simulink model "Quad_Joystick"  (R2018a)
settings: Solver=ode45  StartTime=0.0  StopTime=inf  RelTol=1e-3
undefined symbols (not defined in the file or in its folder): Q
libraries: vrlib x4, realtime_pacer_lib x1, sharedtransform x1
settings Model: Creator=Jarvis  LastModifiedBy=Jarvis

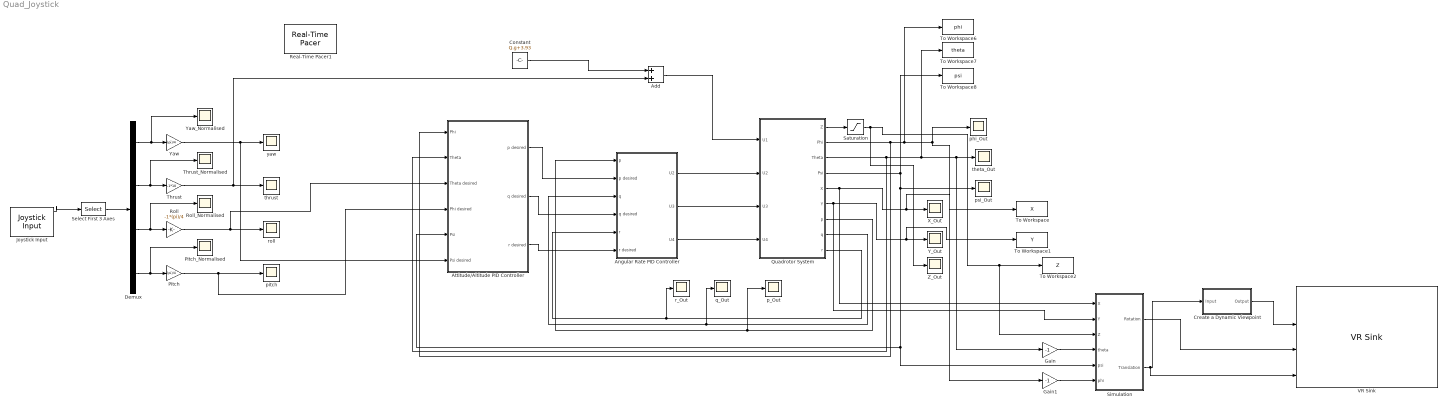
== system Quad_Joystick ==
  Add : Sum
  Angular Rate PID Controller : Subsystem
  Attitude/Altitude PID Controller : Subsystem
  Constant : Constant  Value=Q.g+3.93
  Create a Dynamic Viewpoint : Subsystem
  Demux : Demux
  Gain : Gain  Gain=-1
  Gain1 : Gain  Gain=-1
  Joystick Input : vrlib/Joystick Input  joyid=1  adjustports=on  forcefeed=off
      settings: SourceProductBaseCode=VR
  Pitch : Gain  Gain=(pi)/4
  Pitch_Normalised : Scope
  Quadrotor System : Subsystem
  Real-Time Pacer1 : realtime_pacer_lib/Real-Time Pacer  simTimePerRealTime=1
  Roll : Gain  Gain=-1*(pi)/4
  Roll_Normalised : Scope
  Saturation : Saturate  UpperLimit=100  LowerLimit=0
  Select First 3 Axes : Selector  InputPortWidth=5  IndexOptions=Index vector (dialog)  Indices=[1 2 3 4]  OutputSizes=1
      settings: AttributesFormatString=(Joystick - dependent)
  Simulation : Subsystem
  Thrust : Gain  Gain=-1*10
  Thrust_Normalised : Scope
  To Workspace : ToWorkspace  VariableName=X  SaveFormat=Timeseries  SampleTime=-1
  To Workspace1 : ToWorkspace  VariableName=Y  SaveFormat=Timeseries  SampleTime=-1
  To Workspace2 : ToWorkspace  VariableName=Z  SaveFormat=Timeseries  SampleTime=-1
  To Workspace6 : ToWorkspace  VariableName=phi  SaveFormat=Timeseries  SampleTime=-1
  To Workspace7 : ToWorkspace  VariableName=theta  SaveFormat=Timeseries  SampleTime=-1
  To Workspace8 : ToWorkspace  VariableName=psi  SaveFormat=Timeseries  SampleTime=-1
  VR Sink : vrlib/VR Sink  InstantiateOnLoad=on  SampleTime=0.04  ViewEnable=on  RemoteChange=off  RemoteView=off  FieldsWritten=Flying_(Viewpoint).orientation.4.1.1.double#Flying_(Viewpoint).position.3.1.1.double#QuadCopter.rotation.4.1.1.double#QuadCopter.translation.3.1.1.double  WorldFileName=D:\Projects\Quadcopter\MATLAB\Quad_Simulations\Quad_Simulations\3D QuadCopter\QuadRotor.wrl  AutoView=off  VideoDimensions=[]  AllowVariableSize=off
      settings: SourceProductBaseCode=VR
  X_Out : Scope
  Y_Out : Scope
  Yaw : Gain  Gain=(pi)/4
  Yaw_Normalised : Scope
  Z_Out : Scope
  p_Out : Scope
  phi_Out : Scope
  pitch : Scope
  psi_Out : Scope
  q_Out : Scope
  r_Out : Scope
  roll : Scope
  theta_Out : Scope
  thrust : Scope
  yaw : Scope
  wires:
  Joystick Input/1 -> Select First 3 Axes/1
  Select First 3 Axes/1 -> Demux/1
  Demux/4 -> Pitch_Normalised/1, Pitch/1
  Demux/3 -> Roll_Normalised/1, Roll/1
  Demux/2 -> Thrust_Normalised/1, Thrust/1
  Demux/1 -> Yaw_Normalised/1, Yaw/1
  Yaw/1 -> Attitude/Altitude PID Controller/6(Psi desired), yaw/1
  Roll/1 -> Attitude/Altitude PID Controller/3(Theta desired), roll/1
  Pitch/1 -> Attitude/Altitude PID Controller/4(Phi desired), pitch/1
  Attitude/Altitude PID Controller/3(r desired) -> Angular Rate PID Controller/6(r desired)
  Attitude/Altitude PID Controller/1(p desired) -> Angular Rate PID Controller/2(p desired)
  Quadrotor System/7(p) -> p_Out/1, Angular Rate PID Controller/1(p)
  Quadrotor System/9(r) -> r_Out/1, Angular Rate PID Controller/5(r)
  Quadrotor System/8(q) -> q_Out/1, Angular Rate PID Controller/3(q)
  Angular Rate PID Controller/3(U4) -> Quadrotor System/4(U4)
  Quadrotor System/2(Phi) -> To Workspace6/1, Gain1/1, phi_Out/1, Attitude/Altitude PID Controller/1(Phi)
  Attitude/Altitude PID Controller/2(q desired) -> Angular Rate PID Controller/4(q desired)
  Angular Rate PID Controller/2(U3) -> Quadrotor System/3(U3)
  Angular Rate PID Controller/1(U2) -> Quadrotor System/2(U2)
  Quadrotor System/6(Y) -> Simulation/2(Y), To Workspace1/1, Y_Out/1
  Quadrotor System/4(Psi) -> To Workspace8/1, Simulation/5(psi), Attitude/Altitude PID Controller/5(Psi), psi_Out/1
  Quadrotor System/5(X) -> Simulation/1(X), To Workspace/1, X_Out/1
  Thrust/1 -> Add/2, thrust/1
  Quadrotor System/1(Z) -> Saturation/1
  Saturation/1 -> Z_Out/1, Simulation/3(Z), To Workspace2/1
  Constant/1 -> Add/1
  Add/1 -> Quadrotor System/1(U1)
  Quadrotor System/3(Theta) -> To Workspace7/1, Gain/1, theta_Out/1, Attitude/Altitude PID Controller/2(Theta)
  Gain/1 -> Simulation/4(theta)
  Gain1/1 -> Simulation/6(phi)
  Simulation/2(Translation) -> VR Sink/4, Create a Dynamic Viewpoint/1(Input)
  Create a Dynamic Viewpoint/1(Output) -> VR Sink/2
  Simulation/1(Rotation) -> VR Sink/3

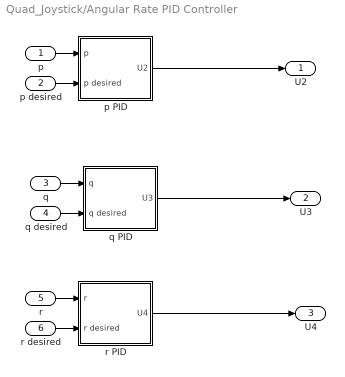
== system Quad_Joystick/Angular Rate PID Controller ==
  p : Inport
  p desired : Inport  Port=2
  q : Inport  Port=3
  q desired : Inport  Port=4
  r : Inport  Port=5
  r desired : Inport  Port=6
  p PID : Subsystem
  q PID : Subsystem
  r PID : Subsystem
  U2 : Outport
  U3 : Outport  Port=2
  U4 : Outport  Port=3
  wires:
  p PID/1(U2) -> U2/1
  q PID/1(U3) -> U3/1
  r PID/1(U4) -> U4/1
  p/1 -> p PID/1(p)
  p desired/1 -> p PID/2(p desired)
  q/1 -> q PID/1(q)
  q desired/1 -> q PID/2(q desired)
  r/1 -> r PID/1(r)
  r desired/1 -> r PID/2(r desired)

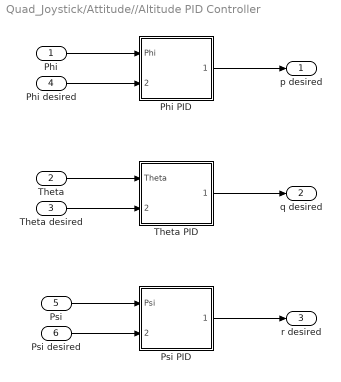
== system Quad_Joystick/Attitude//Altitude PID Controller ==
  Phi : Inport
  Theta : Inport  Port=2
  Theta desired : Inport  Port=3
  Phi desired : Inport  Port=4
  Psi : Inport  Port=5
  Psi desired : Inport  Port=6
  Phi PID : Subsystem
  Psi PID : Subsystem
  Theta PID : Subsystem
  p desired : Outport
  q desired : Outport  Port=2
  r desired : Outport  Port=3
  wires:
  Phi desired/1 -> Phi PID/2(Phi desired)
  Phi/1 -> Phi PID/1(Phi)
  Psi desired/1 -> Psi PID/2(Psi desired)
  Psi/1 -> Psi PID/1(Psi)
  Theta desired/1 -> Theta PID/2(Theta desired)
  Theta/1 -> Theta PID/1(Theta)
  Phi PID/1(p desired) -> p desired/1
  Psi PID/1(r desired) -> r desired/1
  Theta PID/1(q desired) -> q desired/1

== system Quad_Joystick/Create a Dynamic Viewpoint ==
  Input : Inport
  Add1 : Sum
  Add2 : Sum
  Constant1 : Constant  Value=6
  Constant2 : Constant  Value=20
  Demux1 : Demux  Outputs=3
  Mux : Mux  Inputs=3
  Output : Outport
  wires:
  Constant1/1 -> Add1/2
  Add1/1 -> Mux/2
  Constant2/1 -> Add2/2
  Mux/1 -> Output/1
  Demux1/1 -> Mux/1
  Demux1/2 -> Add1/1
  Demux1/3 -> Add2/1
  Add2/1 -> Mux/3
  Input/1 -> Demux1/1

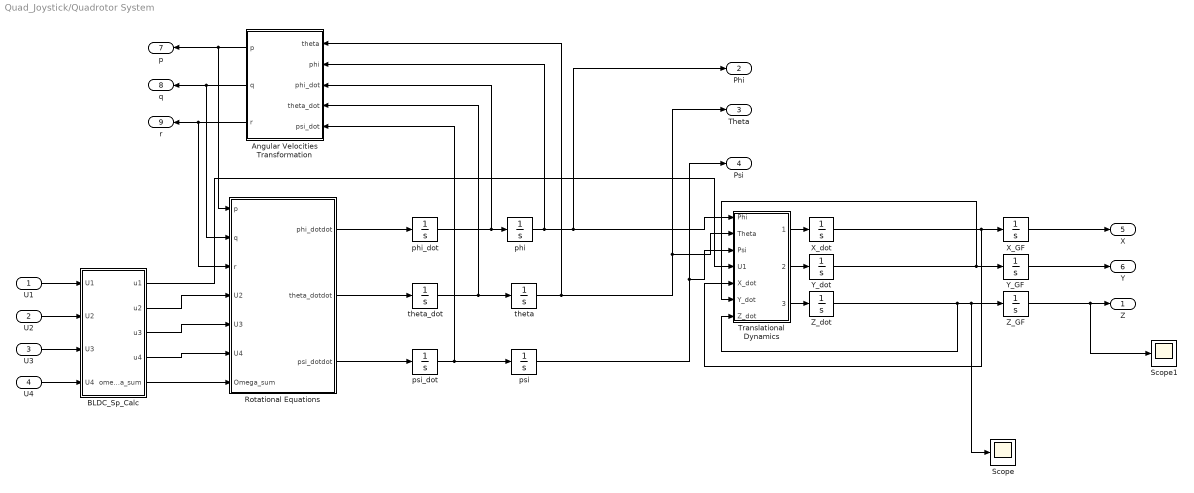
== system Quad_Joystick/Quadrotor System ==
  U1 : Inport
  U2 : Inport  Port=2
  U3 : Inport  Port=3
  U4 : Inport  Port=4
  Angular Velocities Transformation : Subsystem
  BLDC_Sp_Calc : Subsystem
  Rotational Equations : Subsystem
  Scope : Scope
  Scope1 : Scope
  Translational Dynamics : Subsystem
  X_GF : Integrator
  X_dot : Integrator
  Y_GF : Integrator
  Y_dot : Integrator
  Z_GF : Integrator
  Z_dot : Integrator
  phi : Integrator  ZeroCross=off
  phi_dot : Integrator
  psi : Integrator  ZeroCross=off
  psi_dot : Integrator  ZeroCross=off
  theta : Integrator  ZeroCross=off
  theta_dot : Integrator  ZeroCross=off
  Z : Outport
  Phi : Outport  Port=2
  Theta : Outport  Port=3
  Psi : Outport  Port=4
  X : Outport  Port=5
  Y : Outport  Port=6
  p : Outport  Port=7
  q : Outport  Port=8
  r : Outport  Port=9
  wires:
  U1/1 -> BLDC_Sp_Calc/1(U1)
  Angular Velocities Transformation/3(r) -> r/1, Rotational Equations/3(r)
  Angular Velocities Transformation/2(q) -> q/1, Rotational Equations/2(q)
  Angular Velocities Transformation/1(p) -> p/1, Rotational Equations/1(p)
  BLDC_Sp_Calc/4(u4) -> Rotational Equations/6(U4)
  BLDC_Sp_Calc/1(u1) -> Translational Dynamics/4(U1)
  BLDC_Sp_Calc/3(u3) -> Rotational Equations/5(U3)
  BLDC_Sp_Calc/2(u2) -> Rotational Equations/4(U2)
  U3/1 -> BLDC_Sp_Calc/3(U3)
  U2/1 -> BLDC_Sp_Calc/2(U2)
  U4/1 -> BLDC_Sp_Calc/4(U4)
  Rotational Equations/1(phi_dotdot) -> phi_dot/1
  Rotational Equations/3(psi_dotdot) -> psi_dot/1
  phi_dot/1 -> Angular Velocities Transformation/3(phi_dot), phi/1
  theta_dot/1 -> Angular Velocities Transformation/4(theta_dot), theta/1
  psi_dot/1 -> Angular Velocities Transformation/5(psi_dot), psi/1
  Y_GF/1 -> Y/1
  X_GF/1 -> X/1
  Translational Dynamics/3(z dotdot) -> Z_dot/1
  Translational Dynamics/2(y dotdot) -> Y_dot/1
  Y_dot/1 -> Translational Dynamics/6(Y_dot), Y_GF/1
  X_dot/1 -> Translational Dynamics/5(X_dot), X_GF/1
  Translational Dynamics/1(x dotdot) -> X_dot/1
  psi/1 -> Psi/1, Translational Dynamics/3(Psi)
  theta/1 -> Angular Velocities Transformation/1(theta), Theta/1, Translational Dynamics/2(Theta)
  phi/1 -> Angular Velocities Transformation/2(phi), Phi/1, Translational Dynamics/1(Phi)
  BLDC_Sp_Calc/5(omega_sum) -> Rotational Equations/7(Omega_sum)
  Rotational Equations/2(theta_dotdot) -> theta_dot/1
  Z_GF/1 -> Scope1/1, Z/1
  Z_dot/1 -> Translational Dynamics/7(Z_dot), Z_GF/1, Scope/1

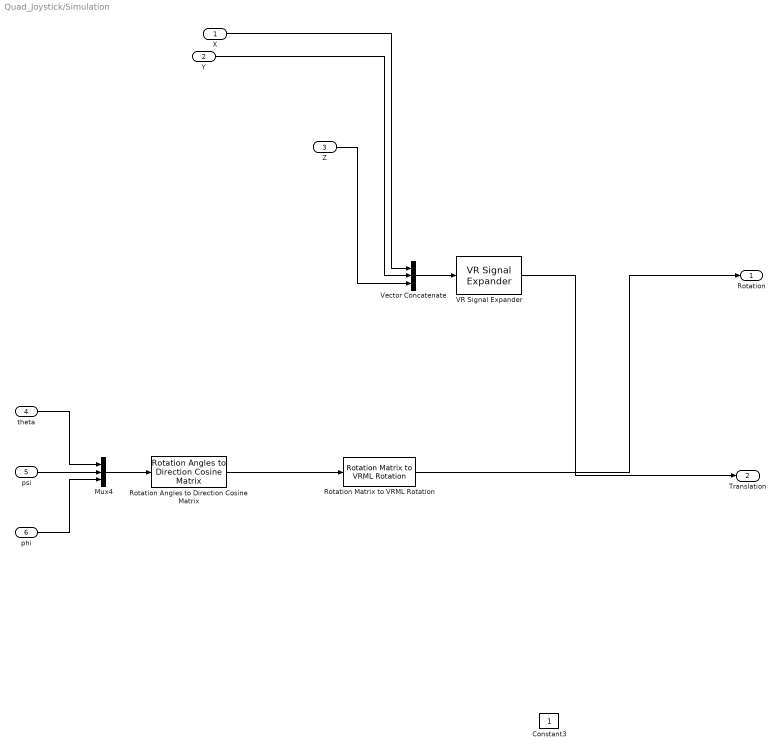
== system Quad_Joystick/Simulation ==
  X : Inport
  Y : Inport  Port=2
  Z : Inport  Port=3
  theta : Inport  Port=4
  psi : Inport  Port=5
  phi : Inport  Port=6
  Constant3 : Constant
  Mux4 : Mux  Inputs=3
  Rotation Angles to Direction Cosine Matrix : sharedtransform/Rotation Angles to Direction Cosine Matrix  rotationOrder=ZYX  aMode=aMode
      settings: SourceProductBaseCode=AE
  Rotation Matrix to VRML Rotation : vrlib/Utilities/Rotation Matrix to VRML Rotation  maxzero=1e-12
      settings: SourceProductName=Simulink 3D Animation  SourceProductBaseCode=VR
  VR Signal Expander : vrlib/VR Signal Expander  outwidth=3  outidx=[1 3 2]
      settings: SourceProductName=Simulink 3D Animation  SourceProductBaseCode=VR
  Vector Concatenate : Concatenate  NumInputs=3
  Rotation : Outport
  Translation : Outport  Port=2
  wires:
  Vector Concatenate/1 -> VR Signal Expander/1
  Z/1 -> Vector Concatenate/3
  Y/1 -> Vector Concatenate/2
  X/1 -> Vector Concatenate/1
  theta/1 -> Mux4/1
  psi/1 -> Mux4/2
  phi/1 -> Mux4/3
  Mux4/1 -> Rotation Angles to Direction Cosine Matrix/1
  Rotation Angles to Direction Cosine Matrix/1 -> Rotation Matrix to VRML Rotation/1
  Rotation Matrix to VRML Rotation/1 -> Rotation/1
  VR Signal Expander/1 -> Translation/1

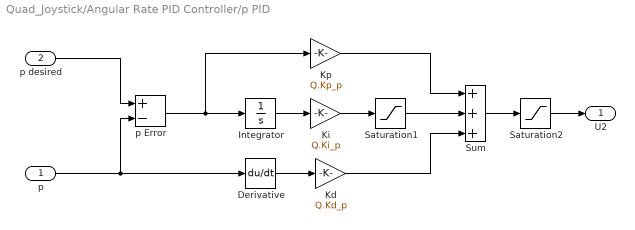
== system Quad_Joystick/Angular Rate PID Controller/p PID ==
  p : Inport
  p desired : Inport  Port=2
  Derivative : Derivative
  Integrator : Integrator
  Kd : Gain  Gain=Q.Kd_p
  Ki : Gain  Gain=Q.Ki_p
  Kp : Gain  Gain=Q.Kp_p
  Saturation1 : Saturate  UpperLimit=Q.U2_max  LowerLimit=Q.U2_min  ZeroCross=off
  Saturation2 : Saturate  UpperLimit=Q.U2_max  LowerLimit=Q.U2_min  ZeroCross=off
  Sum : Sum  Inputs=+++
  p Error : Sum  Inputs=+-
  U2 : Outport
  wires:
  p/1 -> p Error/2, Derivative/1
  p desired/1 -> p Error/1
  Derivative/1 -> Kd/1
  Kp/1 -> Sum/1
  p Error/1 -> Integrator/1, Kp/1
  Integrator/1 -> Ki/1
  Kd/1 -> Sum/3
  Ki/1 -> Saturation1/1
  Saturation1/1 -> Sum/2
  Sum/1 -> Saturation2/1
  Saturation2/1 -> U2/1

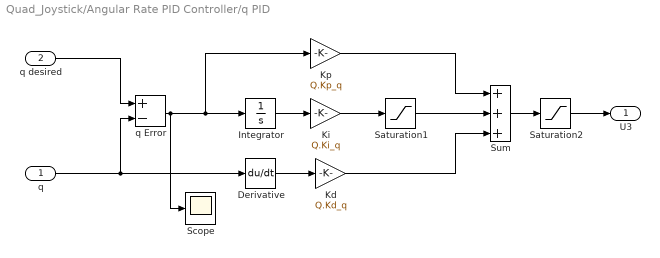
== system Quad_Joystick/Angular Rate PID Controller/q PID ==
  q : Inport
  q desired : Inport  Port=2
  Derivative : Derivative
  Integrator : Integrator
  Kd : Gain  Gain=Q.Kd_q
  Ki : Gain  Gain=Q.Ki_q
  Kp : Gain  Gain=Q.Kp_q
  Saturation1 : Saturate  UpperLimit=Q.U3_max  LowerLimit=Q.U3_min  ZeroCross=off
  Saturation2 : Saturate  UpperLimit=Q.U3_max  LowerLimit=Q.U3_min  ZeroCross=off
  Scope : Scope
  Sum : Sum  Inputs=+++
  q Error : Sum  Inputs=+-
  U3 : Outport
  wires:
  q/1 -> q Error/2, Derivative/1
  q desired/1 -> q Error/1
  Derivative/1 -> Kd/1
  Kp/1 -> Sum/1
  q Error/1 -> Integrator/1, Kp/1, Scope/1
  Integrator/1 -> Ki/1
  Kd/1 -> Sum/3
  Ki/1 -> Saturation1/1
  Saturation1/1 -> Sum/2
  Saturation2/1 -> U3/1
  Sum/1 -> Saturation2/1

== system Quad_Joystick/Angular Rate PID Controller/r PID ==
  r : Inport
  r desired : Inport  Port=2
  Derivative : Derivative
  Integrator : Integrator
  Kd : Gain  Gain=Q.Kd_r
  Ki : Gain  Gain=Q.Ki_r
  Kp : Gain  Gain=Q.Kp_r
  Saturation : Saturate  UpperLimit=Q.U4_max  LowerLimit=Q.U4_min  ZeroCross=off
  Saturation1 : Saturate  UpperLimit=Q.U4_max  LowerLimit=Q.U4_min  ZeroCross=off
  Sum : Sum  Inputs=+++
  r Error : Sum  Inputs=+-
  U4 : Outport
  wires:
  r/1 -> r Error/2, Derivative/1
  r desired/1 -> r Error/1
  Derivative/1 -> Kd/1
  Kp/1 -> Sum/1
  r Error/1 -> Integrator/1, Kp/1
  Integrator/1 -> Ki/1
  Kd/1 -> Sum/3
  Ki/1 -> Saturation/1
  Saturation/1 -> Sum/2
  Sum/1 -> Saturation1/1
  Saturation1/1 -> U4/1

== system Quad_Joystick/Attitude//Altitude PID Controller/Phi PID ==
  Phi : Inport
  Phi desired : Inport  Port=2
  Derivative : Derivative
  Integrator : Integrator
  Kd : Gain  Gain=Q.Kd_phi
  Ki : Gain  Gain=Q.Ki_phi
  Kp : Gain  Gain=Q.Kp_phi
  Psi Error : Sum  Inputs=+-
  Saturation : Saturate  UpperLimit=Q.p_max  LowerLimit=-Q.p_max  ZeroCross=off
  Saturation1 : Saturate  UpperLimit=Q.p_max  LowerLimit=-Q.p_max  ZeroCross=off
  Sum : Sum  Inputs=+++
  p desired : Outport
  wires:
  Phi/1 -> Psi Error/2, Derivative/1
  Phi desired/1 -> Psi Error/1
  Derivative/1 -> Kd/1
  Kp/1 -> Sum/1
  Psi Error/1 -> Integrator/1, Kp/1
  Integrator/1 -> Ki/1
  Kd/1 -> Sum/3
  Ki/1 -> Saturation/1
  Saturation/1 -> Sum/2
  Sum/1 -> Saturation1/1
  Saturation1/1 -> p desired/1

== system Quad_Joystick/Attitude//Altitude PID Controller/Psi PID ==
  Psi : Inport
  Psi desired : Inport  Port=2
  Derivative : Derivative
  Integrator : Integrator
  Kd : Gain  Gain=Q.Kd_psi
  Ki : Gain  Gain=Q.Ki_psi
  Kp : Gain  Gain=Q.Kp_psi
  Psi Error : Sum  Inputs=+-
  Saturation : Saturate  UpperLimit=Q.r_max  LowerLimit=-Q.r_max  ZeroCross=off
  Saturation1 : Saturate  UpperLimit=Q.r_max  LowerLimit=-Q.r_max  ZeroCross=off
  Sum : Sum  Inputs=+++
  r desired : Outport
  wires:
  Psi/1 -> Psi Error/2, Derivative/1
  Psi desired/1 -> Psi Error/1
  Derivative/1 -> Kd/1
  Kp/1 -> Sum/1
  Psi Error/1 -> Integrator/1, Kp/1
  Integrator/1 -> Ki/1
  Kd/1 -> Sum/3
  Ki/1 -> Saturation/1
  Saturation/1 -> Sum/2
  Sum/1 -> Saturation1/1
  Saturation1/1 -> r desired/1

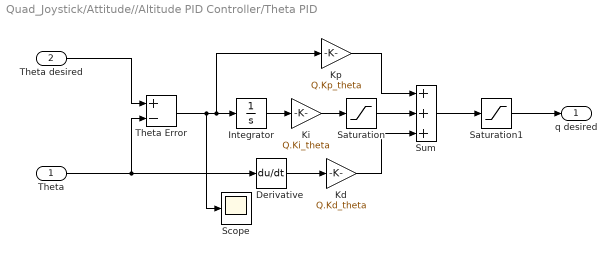
== system Quad_Joystick/Attitude//Altitude PID Controller/Theta PID ==
  Theta : Inport
  Theta desired : Inport  Port=2
  Derivative : Derivative
  Integrator : Integrator
  Kd : Gain  Gain=Q.Kd_theta
  Ki : Gain  Gain=Q.Ki_theta
  Kp : Gain  Gain=Q.Kp_theta
  Saturation : Saturate  UpperLimit=Q.q_max  LowerLimit=-Q.q_max  ZeroCross=off
  Saturation1 : Saturate  UpperLimit=Q.q_max  LowerLimit=-Q.q_max  ZeroCross=off
  Scope : Scope
  Sum : Sum  Inputs=+++
  Theta Error : Sum  Inputs=+-
  q desired : Outport
  wires:
  Theta/1 -> Theta Error/2, Derivative/1
  Theta desired/1 -> Theta Error/1
  Derivative/1 -> Kd/1
  Kp/1 -> Sum/1
  Theta Error/1 -> Integrator/1, Kp/1, Scope/1
  Integrator/1 -> Ki/1
  Kd/1 -> Sum/3
  Ki/1 -> Saturation/1
  Saturation/1 -> Sum/2
  Sum/1 -> Saturation1/1
  Saturation1/1 -> q desired/1

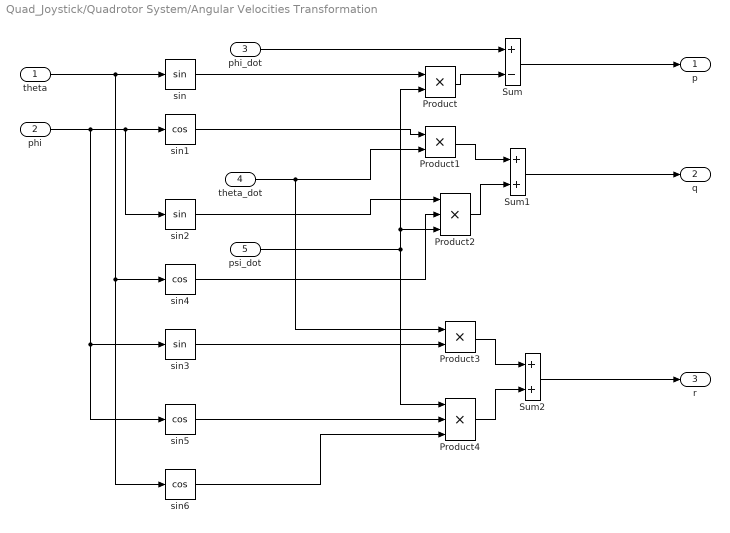
== system Quad_Joystick/Quadrotor System/Angular Velocities Transformation ==
  theta : Inport
  phi : Inport  Port=2
  phi_dot : Inport  Port=3
  theta_dot : Inport  Port=4
  psi_dot : Inport  Port=5
  Product : Product  RndMeth=Zero
  Product1 : Product  RndMeth=Zero
  Product2 : Product  Inputs=3  RndMeth=Zero
  Product3 : Product  RndMeth=Zero
  Product4 : Product  Inputs=3  RndMeth=Zero
  Sum : Sum  Inputs=+-
  Sum1 : Sum
  Sum2 : Sum
  sin : Trigonometry
  sin{1,4..6} (4 alike) : Trigonometry  Operator=cos
  sin2 : Trigonometry
  sin3 : Trigonometry
  p : Outport
  q : Outport  Port=2
  r : Outport  Port=3
  wires:
  Sum2/1 -> r/1
  Sum1/1 -> q/1
  Sum/1 -> p/1
  Product4/1 -> Sum2/2
  Product3/1 -> Sum2/1
  sin6/1 -> Product4/3
  sin5/1 -> Product4/2
  sin3/1 -> Product3/2
  Product2/1 -> Sum1/2
  sin4/1 -> Product2/2
  sin2/1 -> Product2/1
  Product1/1 -> Sum1/1
  theta_dot/1 -> Product3/1, Product1/2
  sin1/1 -> Product1/1
  phi/1 -> sin5/1, sin3/1, sin2/1, sin1/1
  Product/1 -> Sum/2
  psi_dot/1 -> Product4/1, Product2/3, Product/2
  sin/1 -> Product/1
  theta/1 -> sin/1, sin6/1, sin4/1
  phi_dot/1 -> Sum/1

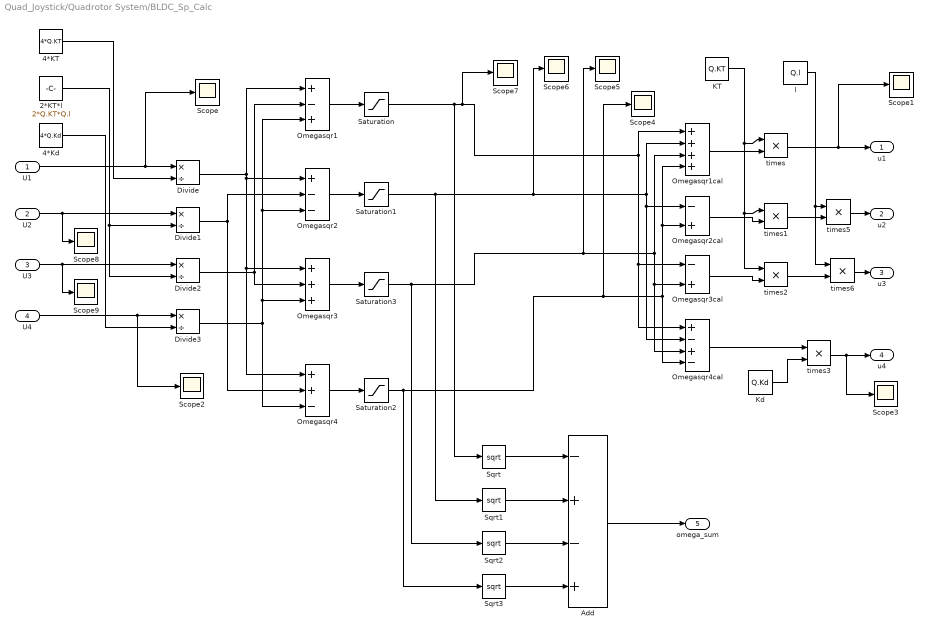
== system Quad_Joystick/Quadrotor System/BLDC_Sp_Calc ==
  U1 : Inport
  U2 : Inport  Port=2
  U3 : Inport  Port=3
  U4 : Inport  Port=4
  2*KT*l : Constant  Value=2*Q.KT*Q.l
  4*KT : Constant  Value=4*Q.KT
  4*Kd : Constant  Value=4*Q.Kd
  Add : Sum  Inputs=-+-+
  Divide{,1..3} (4 alike) : Product  Inputs=*/
  KT : Constant  Value=Q.KT
  Kd : Constant  Value=Q.Kd
  Omegasqr1 : Sum  Inputs=+-+
  Omegasqr1cal : Sum  Inputs=++++
  Omegasqr2 : Sum  Inputs=+--
  Omegasqr2cal : Sum  Inputs=-+
  Omegasqr3 : Sum  Inputs=+++
  Omegasqr3cal : Sum  Inputs=-+
  Omegasqr4 : Sum  Inputs=++-
  Omegasqr4cal : Sum  Inputs=+-+-
  Saturation{,1..3} (4 alike) : Saturate  UpperLimit=Q.max_motor_speed^2  LowerLimit=Q.min_motor_speed^2  ZeroCross=off
  Scope{,1..9} (10 alike) : Scope
  Sqrt{,1..3} (4 alike) : Sqrt  SaturateOnIntegerOverflow=on
  l : Constant  Value=Q.l
  times{,1..3,5..6} (6 alike) : Product  Inputs=**
  u1 : Outport
  u2 : Outport  Port=2
  u3 : Outport  Port=3
  u4 : Outport  Port=4
  omega_sum : Outport  Port=5
  wires:
  Add/1 -> omega_sum/1
  Sqrt3/1 -> Add/4
  Sqrt2/1 -> Add/3
  Sqrt1/1 -> Add/2
  Sqrt/1 -> Add/1
  Omegasqr4/1 -> Saturation2/1
  Omegasqr3/1 -> Saturation3/1
  Omegasqr2/1 -> Saturation1/1
  Omegasqr1/1 -> Saturation/1
  Saturation1/1 -> Scope6/1, Omegasqr4cal/2, Omegasqr2cal/1, Omegasqr1cal/2, Sqrt1/1
  Saturation3/1 -> Scope5/1, Omegasqr4cal/3, Omegasqr3cal/2, Omegasqr1cal/3, Sqrt2/1
  Saturation2/1 -> Scope4/1, Omegasqr4cal/4, Omegasqr2cal/2, Omegasqr1cal/4, Sqrt3/1
  Saturation/1 -> Scope7/1, Omegasqr4cal/1, Omegasqr3cal/1, Omegasqr1cal/1, Sqrt/1
  times2/1 -> times6/2
  times1/1 -> times5/2
  l/1 -> times6/1, times5/1
  times6/1 -> u3/1
  times5/1 -> u2/1
  times3/1 -> Scope3/1, u4/1
  times/1 -> Scope1/1, u1/1
  Kd/1 -> times3/2
  Omegasqr4cal/1 -> times3/1
  Omegasqr3cal/1 -> times2/2
  Omegasqr2cal/1 -> times1/2
  Omegasqr1cal/1 -> times/2
  KT/1 -> times2/1, times1/1, times/1
  Divide1/1 -> Omegasqr4/2, Omegasqr2/2
  Divide3/1 -> Omegasqr4/3, Omegasqr3/3, Omegasqr2/3, Omegasqr1/3
  Divide2/1 -> Omegasqr3/2, Omegasqr1/2
  Divide/1 -> Omegasqr4/1, Omegasqr3/1, Omegasqr2/1, Omegasqr1/1
  4*Kd/1 -> Divide3/2
  U4/1 -> Scope2/1, Divide3/1
  U3/1 -> Scope9/1, Divide2/1
  2*KT*l/1 -> Divide2/2, Divide1/2
  U2/1 -> Scope8/1, Divide1/1
  4*KT/1 -> Divide/2
  U1/1 -> Scope/1, Divide/1

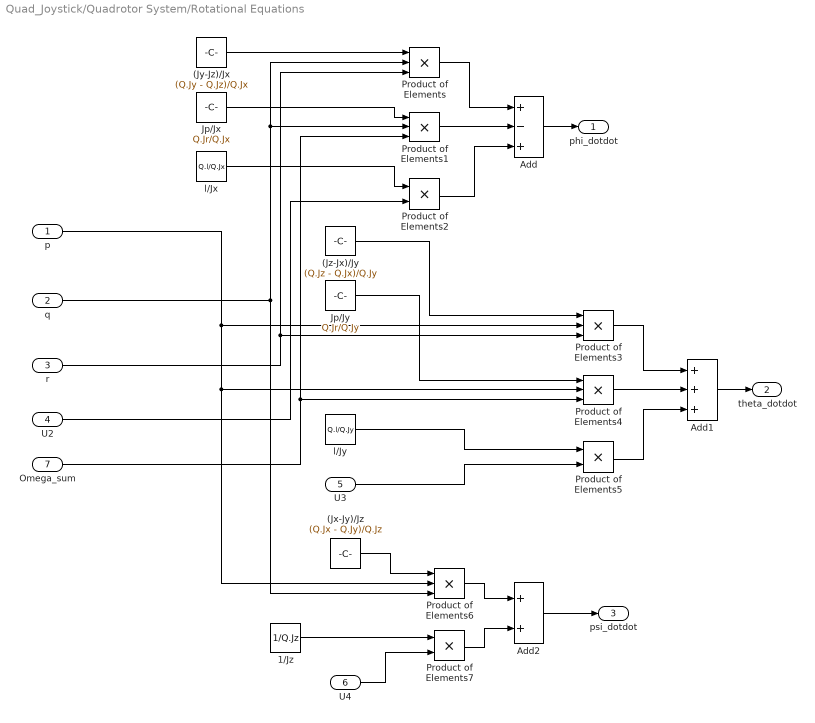
== system Quad_Joystick/Quadrotor System/Rotational Equations ==
  p : Inport
  q : Inport  Port=2
  r : Inport  Port=3
  U2 : Inport  Port=4
  U3 : Inport  Port=5
  U4 : Inport  Port=6
  Omega_sum : Inport  Port=7
  (Jx-Jy)/Jz : Constant  Value=(Q.Jx - Q.Jy)/Q.Jz
  (Jy-Jz)/Jx : Constant  Value=(Q.Jy - Q.Jz)/Q.Jx
  (Jz-Jx)/Jy : Constant  Value=(Q.Jz - Q.Jx)/Q.Jy
  1/Jz : Constant  Value=1/Q.Jz
  Add : Sum  Inputs=+-+
  Add1 : Sum  Inputs=+++
  Add2 : Sum
  Jp/Jx : Constant  Value=Q.Jr/Q.Jx
  Jp/Jy : Constant  Value=Q.Jr/Q.Jy
  Product of Elements{,1,3..4,6} (5 alike) : Product  Inputs=3
  Product of Elements2 : Product
  Product of Elements5 : Product
  Product of Elements7 : Product
  l/Jx : Constant  Value=Q.l/Q.Jx
  l/Jy : Constant  Value=Q.l/Q.Jy
  phi_dotdot : Outport
  theta_dotdot : Outport  Port=2
  psi_dotdot : Outport  Port=3
  wires:
  Product of Elements6/1 -> Add2/1
  (Jx-Jy)/Jz/1 -> Product of Elements6/1
  1/Jz/1 -> Product of Elements7/1
  U4/1 -> Product of Elements7/2
  Add2/1 -> psi_dotdot/1
  Product of Elements7/1 -> Add2/2
  p/1 -> Product of Elements6/2, Product of Elements4/2, Product of Elements3/2
  U3/1 -> Product of Elements5/2
  l/Jy/1 -> Product of Elements5/1
  Jp/Jy/1 -> Product of Elements4/1
  (Jz-Jx)/Jy/1 -> Product of Elements3/1
  Add1/1 -> theta_dotdot/1
  Product of Elements5/1 -> Add1/3
  Product of Elements4/1 -> Add1/2
  Product of Elements3/1 -> Add1/1
  Omega_sum/1 -> Product of Elements4/3, Product of Elements1/3
  U2/1 -> Product of Elements2/2
  l/Jx/1 -> Product of Elements2/1
  Jp/Jx/1 -> Product of Elements1/1
  r/1 -> Product of Elements3/3, Product of Elements/3
  q/1 -> Product of Elements6/3, Product of Elements1/2, Product of Elements/2
  (Jy-Jz)/Jx/1 -> Product of Elements/1
  Add/1 -> phi_dotdot/1
  Product of Elements2/1 -> Add/3
  Product of Elements1/1 -> Add/2
  Product of Elements/1 -> Add/1

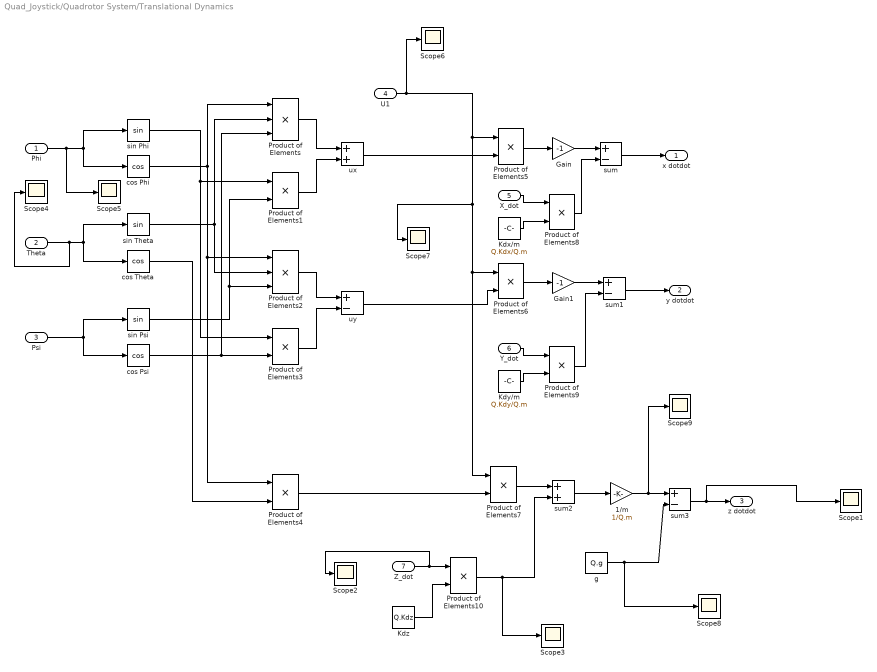
== system Quad_Joystick/Quadrotor System/Translational Dynamics ==
  Phi : Inport
  Theta : Inport  Port=2
  Psi : Inport  Port=3
  U1 : Inport  Port=4
  X_dot : Inport  Port=5
  Y_dot : Inport  Port=6
  Z_dot : Inport  Port=7
  1/m : Gain  Gain=1/Q.m
  Gain : Gain  Gain=-1
  Gain1 : Gain  Gain=-1
  Kdx/m : Constant  Value=Q.Kdx/Q.m
  Kdy/m : Constant  Value=Q.Kdy/Q.m
  Kdz : Constant  Value=Q.Kdz
  Product of Elements : Product  Inputs=3
  Product of Elements{1,3..10} (9 alike) : Product
  Product of Elements2 : Product  Inputs=3
  Scope{1..9} (9 alike) : Scope
  cos Phi : Trigonometry  Operator=cos
  cos Psi : Trigonometry  Operator=cos
  cos Theta : Trigonometry  Operator=cos
  g : Constant  Value=Q.g
  sin Phi : Trigonometry
  sin Psi : Trigonometry
  sin Theta : Trigonometry
  sum : Sum  Inputs=+-
  sum1 : Sum  Inputs=+-
  sum2 : Sum
  sum3 : Sum  Inputs=+-
  ux : Sum
  uy : Sum  Inputs=+-
  x dotdot : Outport
  y dotdot : Outport  Port=2
  z dotdot : Outport  Port=3
  wires:
  sum1/1 -> y dotdot/1
  Product of Elements9/1 -> sum1/2
  Gain1/1 -> sum1/1
  Kdy/m/1 -> Product of Elements9/2
  Y_dot/1 -> Product of Elements9/1
  sum/1 -> x dotdot/1
  Product of Elements8/1 -> sum/2
  Gain/1 -> sum/1
  Kdx/m/1 -> Product of Elements8/2
  X_dot/1 -> Product of Elements8/1
  Product of Elements6/1 -> Gain1/1
  Product of Elements5/1 -> Gain/1
  U1/1 -> Scope7/1, Product of Elements7/1, Product of Elements6/1, Product of Elements5/1, Scope6/1
  Product of Elements4/1 -> Product of Elements7/2
  cos Theta/1 -> Product of Elements4/2
  uy/1 -> Product of Elements6/2
  Product of Elements3/1 -> uy/2
  Product of Elements2/1 -> uy/1
  ux/1 -> Product of Elements5/2
  Product of Elements1/1 -> ux/2
  Product of Elements/1 -> ux/1
  sin Psi/1 -> Product of Elements2/3, Product of Elements1/2
  sin Phi/1 -> Product of Elements3/1, Product of Elements1/1
  cos Phi/1 -> Product of Elements4/1, Product of Elements2/1, Product of Elements/1
  cos Psi/1 -> Product of Elements3/2, Product of Elements/3
  sin Theta/1 -> Product of Elements2/2, Product of Elements/2
  Psi/1 -> cos Psi/1, sin Psi/1
  Theta/1 -> Scope4/1, cos Theta/1, sin Theta/1
  Phi/1 -> Scope5/1, cos Phi/1, sin Phi/1
  Product of Elements7/1 -> sum2/1
  Z_dot/1 -> Scope2/1, Product of Elements10/1
  Kdz/1 -> Product of Elements10/2
  Product of Elements10/1 -> Scope3/1, sum2/2
  sum2/1 -> 1/m/1
  1/m/1 -> Scope9/1, sum3/1
  g/1 -> Scope8/1, sum3/2
  sum3/1 -> Scope1/1, z dotdot/1
